simulink model "controller_attitude_roll"  (R2021a)
settings: Solver=FixedStepAuto  StartTime=0.0  StopTime=10.0  FixedStep=1/sim_freq  RelTol=1e-3
undefined symbols (not defined in the file): G_R_OL_DENOM, G_R_OL_NUM, K_phi, sim_freq
settings Model: Creator=francois  LastModifiedBy=esl
settings SolverCC: AlgebraicLoopSolver=TrustRegion
settings DebuggingCC: SFMachineParentedDataDiag=warning

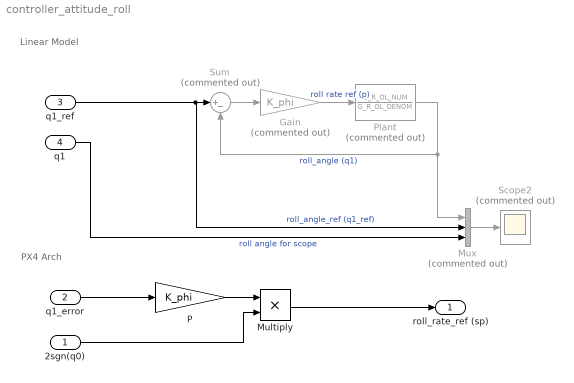
== system controller_attitude_roll ==
  note: Linear Model
  note: PX4 Arch
  2sgn(q0) : Inport
  q1_error : Inport  Port=2
  q1_ref : Inport  Port=3
  q1 : Inport  Port=4  SampleTime=1/sim_freq
  Gain : Gain  Commented=on  Gain=K_phi
  Multiply : Product
  Mux : Mux  Commented=on  Inputs=3
  P : Gain  Gain=K_phi
  Plant : TransferFcn  Commented=on  Numerator=G_R_OL_NUM  Denominator=G_R_OL_DENOM
  Scope2 : Scope  Commented=on
  Sum : Sum  Commented=on  Inputs=|+-
  roll_rate_ref (sp) : Outport  VectorParamsAs1DForOutWhenUnconnected=off
  wires:
  q1_ref/1 -> Mux/2, Sum/1  "roll_angle_ref (q1_ref)"
  Plant/1 -> Mux/1, Sum/2  "roll_angle (q1)"
  Sum/1 -> Gain/1
  Gain/1 -> Plant/1  "roll rate ref (p)"
  P/1 -> Multiply/1
  2sgn(q0)/1 -> Multiply/2
  q1_error/1 -> P/1
  Multiply/1 -> roll_rate_ref (sp)/1
  q1/1 -> Mux/3  "roll angle for scope"
  Mux/1 -> Scope2/1
